simulink model "SolarPanel102"  (R2016b)
settings: Solver=VariableStepAuto  StartTime=0.0  StopTime=1  RelTol=1e-3
libraries: powerlib x11, simulink x3
settings Model: Creator=hp  LastModifiedBy=hp

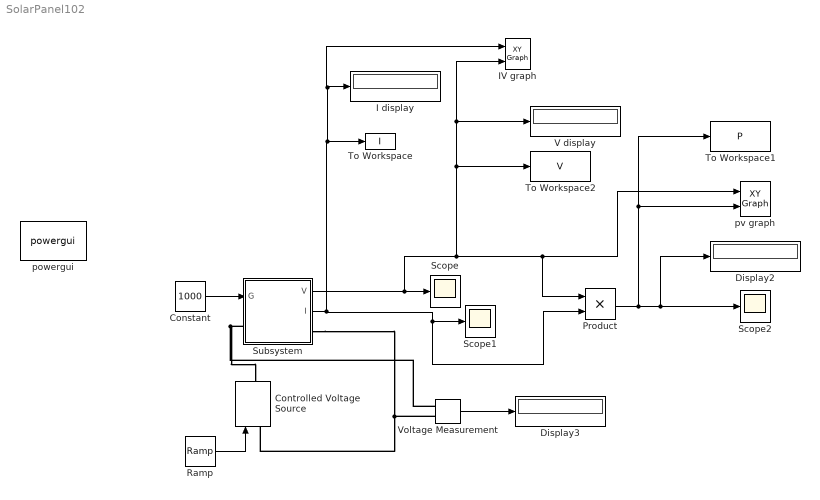
== system SolarPanel102 ==
  Constant : Constant  Value=1000
  Controlled Voltage Source : powerlib/Electrical Sources/Controlled Voltage Source  Initialize=on  Source_Type=AC  Amplitude=0  Phase=0  Frequency=0  Measurements=None
  Display2 : Display
  Display3 : Display
  I display : Display
  IV graph : simulink/Sinks/XY Graph  xmin=-1  xmax=310  ymin=-1  ymax=125000  st=-1
  Product : Product
  Ramp : simulink/Sources/Ramp  slope=306  start=0  X0=0
  Scope : Scope
  Scope1 : Scope
  Scope2 : Scope
  Subsystem : Subsystem  mask{Ns=500, Np=66}
      mask init:
      | V = 1.5;
      | k = 1.3806e-23;
      | T = 298;
      | q = 1.602e-19;
      | Vt = V*k*T/q;
      | Vt_panel = Vt*Ns;
      | Iph=8;
      | Iph_panel=Iph*Np;
      | Io= 9.845e-7;
      | Io_panel=Io*Np;
      | Rs=0.001;
      | Rs_panel=Rs*Ns/Np;
      | Rsh=142.94;
      | Rsh_panel=Rsh*Ns/Np;
      | G0=1000;
  To Workspace : ToWorkspace  VariableName=I  SampleTime=-1
  To Workspace1 : ToWorkspace  VariableName=P  SampleTime=-1
  To Workspace2 : ToWorkspace  VariableName=V  SampleTime=-1
  V display : Display
  Voltage Measurement : powerlib/Measurements/Voltage Measurement  PhasorSimulation=off  OutputType=Complex  PSBequivalent=0
  powergui : powerlib/powergui  Priority=1  SimulationMode=Discrete  SolverType=Tustin/Backward Euler (TBE)  SampleTime=50e-6  frequency=60  SPID=off  DisableSnubberDevices=off  DisableRonSwitches=off  DisableVfSwitches=off  SwTol=0  DisplayEquations=off  Interpol=off  ExternalGateDelay=off  methode=off  Ts=10  FunctionMessages=off  echomessages=off  HookPort=off  EnableUseOfTLC=off  x0status=blocks  frequencyindice=0  Pbase=100e6  ErrMax=1e-4  Iterations=50  UnitsV=kV  UnitsW=MW  buscounter=0  RestoreLinks=warning  ResistiveCurrentMeasurement=off  Frange=[0:2:500]  Ylog=off  Xlog=on  ShowGrid=off  save=off  variable=ZData  structure=0  ZoomFFT=off  StartTime=0.0  cycles=1  DisplayStyle=1  fundamental=60  FreqAxis=off  MaxFrequency=1000  frequencyindicesteady=1  RmsSteady=1  display=off
  "pv graph " : simulink/Sinks/XY Graph  xmin=-50  xmax=900000  ymin=-50  ymax=40000  st=-1
  wires:
  Constant/1 -> Subsystem/1(G)
  Subsystem/1(V) -> To Workspace2/1, IV graph/2, V display/1, "pv graph "/1, Product/1, Scope/1
  Subsystem/2(I) -> IV graph/1, I display/1, To Workspace/1, Product/2, Scope1/1
  Product/1 -> "pv graph "/2, To Workspace1/1, Display2/1, Scope2/1
  Ramp/1 -> Controlled Voltage Source/1
  Voltage Measurement/1 -> Display3/1
  connections:
  Subsystem/LConn1 -- Voltage Measurement/LConn1 -- Controlled Voltage Source/RConn1
  Subsystem/RConn1 -- Voltage Measurement/LConn2 -- Controlled Voltage Source/LConn1

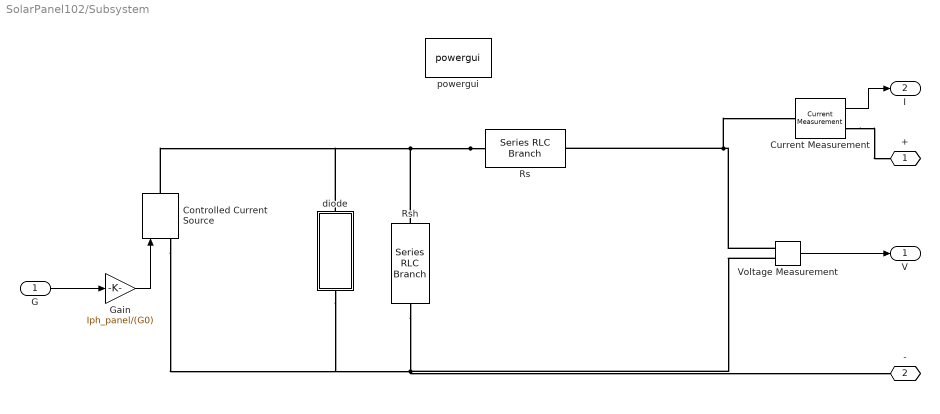
== system SolarPanel102/Subsystem ==
  G : Inport
  Controlled Current Source : powerlib/Electrical Sources/Controlled Current Source  Initialize=on  Source_Type=AC  Amplitude=0  Phase=0  Frequency=0  Measurements=None
  Current Measurement : powerlib/Measurements/Current Measurement  PhasorSimulation=off  OutputType=Complex  PSBequivalent=0
  Gain : Gain  Gain=Iph_panel/(G0)
  Rs : powerlib/Elements/Series RLC Branch  LConnTagsString=__new0  RConnTagsString=__new0  BranchType=R  Resistance=Rs_panel  Inductance=1e-3  SetiL0=off  InitialCurrent=0  Capacitance=1e-6  Setx0=off  InitialVoltage=0  Measurements=None
  Rsh : powerlib/Elements/Series RLC Branch  LConnTagsString=__new0  RConnTagsString=__new0  BranchType=R  Resistance=Rsh_panel  Inductance=1e-3  SetiL0=off  InitialCurrent=0  Capacitance=1e-6  Setx0=off  InitialVoltage=0  Measurements=None
  Voltage Measurement : powerlib/Measurements/Voltage Measurement  PhasorSimulation=off  OutputType=Complex  PSBequivalent=0
  "diode " : Subsystem
  powergui : powerlib/powergui  Priority=1  SimulationMode=Discrete  SolverType=Tustin/Backward Euler (TBE)  SampleTime=50e-6  frequency=60  SPID=off  DisableSnubberDevices=off  DisableRonSwitches=off  DisableVfSwitches=off  SwTol=0  DisplayEquations=off  Interpol=off  ExternalGateDelay=off  methode=off  Ts=10  FunctionMessages=off  echomessages=off  HookPort=off  EnableUseOfTLC=off  x0status=blocks  frequencyindice=60  Pbase=100e6  ErrMax=1e-4  Iterations=50  UnitsV=kV  UnitsW=MW  buscounter=0  RestoreLinks=warning  ResistiveCurrentMeasurement=off  Frange=[0:2:500]  Ylog=off  Xlog=on  ShowGrid=off  save=off  variable=ZData  structure=0  ZoomFFT=off  StartTime=0.0  cycles=1  DisplayStyle=1  fundamental=60  FreqAxis=off  MaxFrequency=1000  frequencyindicesteady=1  RmsSteady=1  display=off
  + : PMIOPort  Port=1  Side=Left
  - : PMIOPort  Port=2  Side=Right
  V : Outport
  I : Outport  Port=2
  wires:
  G/1 -> Gain/1
  Gain/1 -> Controlled Current Source/1
  Voltage Measurement/1 -> V/1
  Current Measurement/1 -> I/1
  connections:
  Rs/LConn1 -- "diode "/LConn1 -- Controlled Current Source/RConn1 -- Rsh/LConn1
  Rsh/RConn1 -- "diode "/RConn1 -- Controlled Current Source/LConn1 -- Voltage Measurement/LConn2 -- -/RConn1
  Voltage Measurement/LConn1 -- Current Measurement/LConn1 -- Rs/RConn1
  Current Measurement/RConn1 -- +/RConn1

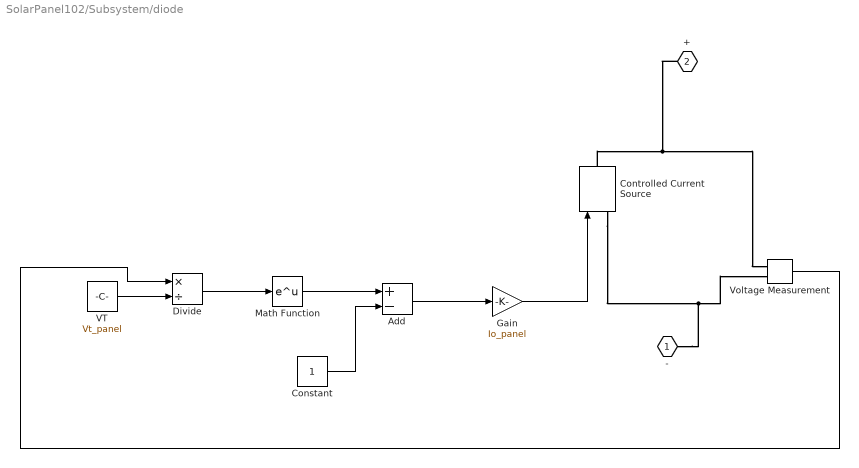
== system SolarPanel102/Subsystem/diode  ==
  Add : Sum  Inputs=+-
  Constant : Constant
  Controlled Current Source : powerlib/Electrical Sources/Controlled Current Source  Initialize=on  Source_Type=AC  Amplitude=0  Phase=0  Frequency=0  Measurements=None
  Divide : Product  Inputs=*/
  Gain : Gain  Gain=Io_panel
  Math Function : Math  SaturateOnIntegerOverflow=on
  VT : Constant  Value=Vt_panel
  Voltage Measurement : powerlib/Measurements/Voltage Measurement  PhasorSimulation=off  OutputType=Complex  PSBequivalent=0
  - : PMIOPort  Port=1  Side=Right
  + : PMIOPort  Port=2  Side=Left
  wires:
  VT/1 -> Divide/2
  Divide/1 -> Math Function/1
  Math Function/1 -> Add/1
  Add/1 -> Gain/1
  Gain/1 -> Controlled Current Source/1
  Constant/1 -> Add/2
  Voltage Measurement/1 -> Divide/1
  connections:
  +/RConn1 -- Voltage Measurement/LConn1 -- Controlled Current Source/RConn1
  -/RConn1 -- Voltage Measurement/LConn2 -- Controlled Current Source/LConn1
